simulink model "Admittace_Control"  (R2020a)
settings: Solver=FixedStepAuto  StartTime=0.0  StopTime=2  FixedStep=0.001  RelTol=1e-3  EnableMultiTasking=on
undefined symbols (not defined in the file or in its folder): X, Y, Z
libraries: sm_lib x79, nesl_utility x41, roblocks x8
(part 3 of 3)

== matlab function Admittace_Control/Exoskeleton/Subsystem/Admittance Control/xd+xe ==
  data: xyzkps0 input; xyzkps output; dxyzkps input
function xyzkps= add_compter(xyzkps0, dxyzkps)

xyzkps = zeros(1,6);
xyzkps(1)=xyzkps0(1)+dxyzkps(1);
xyzkps(2)=xyzkps0(2)+dxyzkps(2);
xyzkps(3)=xyzkps0(3)+dxyzkps(3);
%-------------
rpy=dxyzkps(4:6);
sx=sin(rpy(1));
cx=cos(rpy(1));
sy=sin(rpy(2));
cy=cos(rpy(2));
sz=sin(rpy(3));
cz=cos(rpy(3));
dR=[cy*cz  cz*sx*sy - cx*sz  sx*sz + cx*cz*sy;
	cy*sz  cx*cz + sx*sy*sz  cx*sy*sz - cz*sx;
	 -sy   cy*sx  cx*cy];

%-------------
rpy=xyzkps0(4:6);
sx=sin(rpy(1));
cx=cos(rpy(1));
sy=sin(rpy(2));
cy=cos(rpy(2));
sz=sin(rpy(3));
cz=cos(rpy(3));
R0=[cy*cz  cz*sx*sy - cx*sz  sx*sz + cx*cz*sy;
	cy*sz  cx*cz + sx*sy*sz  cx*sy*sz - cz*sx;
	 -sy   cy*sx  cx*cy];
R=dR*R0;
 
xyzkps(5)= atan2(-R(3,1),sqrt(R(1,1)*R(1,1)+R(2,1)*R(2,1))); 
        if (abs(abs(xyzkps(5)) - pi / 2.0) < 0.0000001)
                if (xyzkps(5) > 0) %pi/2
                    xyzkps(5) = pi / 2.0;
                    xyzkps(6) = 0.0;
                    xyzkps(4) = atan2(R(1,2),R(2,2));
                else%-pi/2
                    xyzkps(5) = -pi / 2.0;
                    xyzkps(6) = 0.0;
                    xyzkps(4) = -atan2(R(1,2), R(2,2));
                end
        else
                cp = cos(xyzkps(5));
                xyzkps(6) = atan2(R(2,1)/cp,R(1,1)/cp);
                xyzkps(4) = atan2(R(3,2)/cp, R(3,3)/cp);
        end


end

== matlab function Admittace_Control/Exoskeleton/Subsystem1/Admittance Control/jacobi ==
  data: Jn_Base input; dx output; dQ input
function dx = fcn(Jn_Base,dQ)
dx = Jn_Base*dQ;

== matlab function Admittace_Control/Exoskeleton/Subsystem1/Admittance Control/vel->pos ==
  data: dxe input; xe input; xe_targ output
function xe_targ   = vel_integral(dxe,xe)
%% parameter
xe_targ=zeros(1,6);
dt = 0.001;
dt_dxe=dxe*dt;
xe_targ(1)=xe(1)+dt_dxe(1);
xe_targ(2)=xe(2)+dt_dxe(2);
xe_targ(3)=xe(3)+dt_dxe(3);

%-----------等效转轴转姿态矩阵----------
eqaxis=dt_dxe(4:6);

A=norm(eqaxis);
if (A>1e-10)
axis=eqaxis./A;
sx=sin(A);cx=cos(A);v=1-cx;
dR=[axis(1)*axis(1)*v + cx	axis(1)*axis(2)*v - axis(3)*sx 	axis(1)*axis(3)*v + axis(2)*sx;
  axis(1)*axis(2)*v + axis(3)*sx 	axis(2)*axis(2)*v + cx 	 axis(2)*axis(3)*v - axis(1)*sx;
  axis(1)*axis(3)*v - axis(2)*sx 	axis(2)*axis(3)*v + axis(1)*sx  axis(3)*axis(3)*v + cx];
else
  dR=[1 0 0;
      0 1 0;
      0 0 1];
end

%-----------等效转轴转姿态矩阵----------
eqaxis=xe(4:6);
A=norm(eqaxis);
if (A>1e-10)
axis=eqaxis./A;
sx=sin(A);cx=cos(A);v=1-cx;
Re=[axis(1)*axis(1)*v + cx	axis(1)*axis(2)*v - axis(3)*sx 	axis(1)*axis(3)*v + axis(2)*sx;
  axis(1)*axis(2)*v + axis(3)*sx 	axis(2)*axis(2)*v + cx 	 axis(2)*axis(3)*v - axis(1)*sx;
  axis(1)*axis(3)*v - axis(2)*sx 	axis(2)*axis(3)*v + axis(1)*sx  axis(3)*axis(3)*v + cx];
else
  Re=[1 0 0;
      0 1 0;
      0 0 1];
end


R=dR*Re;%姿态叠加

%-----------姿态矩阵转固定角----------
xe_targ(5)= atan2(-R(3,1),sqrt(R(1,1)*R(1,1)+R(2,1)*R(2,1))); 
        if (abs(abs(xe_targ(5)) - pi / 2.0) < 0.0000001)
                if (xe_targ(5) > 0) %pi/2
                    xe_targ(5) = pi / 2.0;
                    xe_targ(6) = 0.0;
                    xe_targ(4) = atan2(R(1,2),R(2,2));
                else%-pi/2
                    xe_targ(5) = -pi / 2.0;
                    xe_targ(6) = 0.0;
                    xe_targ(4) = -atan2(R(1,2), R(2,2));
                end
        else
                cp = cos(xe_targ(5));
                xe_targ(6) = atan2(R(2,1)/cp,R(1,1)/cp);
                xe_targ(4) = atan2(R(3,2)/cp, R(3,3)/cp);
        end




end

== matlab function Admittace_Control/Exoskeleton/Subsystem1/Admittance Control/x-xd ==
  data: x input; xd input; xe output
function xe = Change(x,xd)
%% parameter
xe=zeros(1,6);
dt = 0.001;

V1 = [x(1)-xd(1),x(2)-xd(2),x(3)-xd(3) ];

p = x(4);
q = x(5);
r = x(6);
%% output
I= diag(ones(1,3));
%%
sx = sin(p);
cx = cos(p);
sy = sin(q);
cy = cos(q);
sz = sin(r);
cz = cos(r);
I(1,1) = cy*cz;			
I(1,2) = cz*sx*sy - cx*sz;	
I(1,3) = sx*sz + cx*cz*sy;
I(2,1) = cy*sz;	
I(2,2) = cx*cz + sx*sy*sz;			
I(2,3) = cx*sy*sz - cz*sx;
I(3,1) = -sy;	
I(3,2) = cy*sx;	
I(3,3) = cx*cy;

%%
pw = xd(4);
qw = xd(5);
rw = xd(6);
%% output
Iw= diag(ones(1,3));
%%
sxw = sin(pw);
cxw = cos(pw);
syw = sin(qw);
cyw = cos(qw);
szw = sin(rw);
czw = cos(rw);
Iw(1,1) = cyw*czw;			
Iw(1,2) = czw*sxw*syw - cxw*szw;	
Iw(1,3) = sxw*szw + cxw*czw*syw;
Iw(2,1) = cyw*szw;	
Iw(2,2) = cxw*czw + sxw*syw*szw;			
Iw(2,3) = cxw*syw*szw - czw*sxw;
Iw(3,1) = -syw;	
Iw(3,2) = cyw*sxw;	
Iw(3,3) = cxw*cyw;
V2=V1;
DI=I*Iw';
%%转换成等效转轴

cp=(DI(1,1)+DI(2,2)+DI(3,3)-1)/2.0;
if (cp>1-(1e-10))
    V2(1) = 0;
    V2(2) = 0;
    V2(3) = 0;
else
    if (cp<-1+(1e-10))
        V2(1) = sqrt( (DI(1,1)+1.0)/2);
        V2(2) = sqrt( (DI(2,2)+1.0)/2);
        V2(3) = sqrt( (DI(3,3)+1.0)/2);
        if ( DI(1,3)< 0)  
            V2(1) =- V2(1);
        end
        if ( DI(3,2)< 0)  
            V2(2) =- V2(2);
        end
        if (  V2(1)* V2(2)*DI(1,2) < 0)
            V2(1)=- V2(1);  % this last line can be necessary when z is 0
        end
            % z always >= 0
       % if z equal to zero
        V2(1) = V2(1)*pi;
        V2(2) = V2(2)*pi;
        V2(3) = V2(3)*pi;
    else
        Q=acos(cp);

        V2(1) = Q*0.5*(DI(3,2)-DI(2,3))/sin(Q);
        V2(2) = Q*0.5*(DI(1,3)-DI(3,1))/sin(Q);
        V2(3) = Q*0.5*(DI(2,1)-DI(1,2))/sin(Q);
    end
end
xe = [V1,V2];

end

== matlab function Admittace_Control/Exoskeleton/Subsystem1/Admittance Control/xd+xe ==
  data: xyzkps0 input; xyzkps output; dxyzkps input
function xyzkps= add_compter(xyzkps0, dxyzkps)

xyzkps = zeros(1,6);
xyzkps(1)=xyzkps0(1)+dxyzkps(1);
xyzkps(2)=xyzkps0(2)+dxyzkps(2);
xyzkps(3)=xyzkps0(3)+dxyzkps(3);
%-------------
rpy=dxyzkps(4:6);
sx=sin(rpy(1));
cx=cos(rpy(1));
sy=sin(rpy(2));
cy=cos(rpy(2));
sz=sin(rpy(3));
cz=cos(rpy(3));
dR=[cy*cz  cz*sx*sy - cx*sz  sx*sz + cx*cz*sy;
	cy*sz  cx*cz + sx*sy*sz  cx*sy*sz - cz*sx;
	 -sy   cy*sx  cx*cy];

%-------------
rpy=xyzkps0(4:6);
sx=sin(rpy(1));
cx=cos(rpy(1));
sy=sin(rpy(2));
cy=cos(rpy(2));
sz=sin(rpy(3));
cz=cos(rpy(3));
R0=[cy*cz  cz*sx*sy - cx*sz  sx*sz + cx*cz*sy;
	cy*sz  cx*cz + sx*sy*sz  cx*sy*sz - cz*sx;
	 -sy   cy*sx  cx*cy];
R=dR*R0;
 
xyzkps(5)= atan2(-R(3,1),sqrt(R(1,1)*R(1,1)+R(2,1)*R(2,1))); 
        if (abs(abs(xyzkps(5)) - pi / 2.0) < 0.0000001)
                if (xyzkps(5) > 0) %pi/2
                    xyzkps(5) = pi / 2.0;
                    xyzkps(6) = 0.0;
                    xyzkps(4) = atan2(R(1,2),R(2,2));
                else%-pi/2
                    xyzkps(5) = -pi / 2.0;
                    xyzkps(6) = 0.0;
                    xyzkps(4) = -atan2(R(1,2), R(2,2));
                end
        else
                cp = cos(xyzkps(5));
                xyzkps(6) = atan2(R(2,1)/cp,R(1,1)/cp);
                xyzkps(4) = atan2(R(3,2)/cp, R(3,3)/cp);
        end


end

== matlab function Admittace_Control/Exoskeleton/Subsystem1/Admittance Control/Admittance Control ==
  data: dxe input; xe input; ddxe output; Fe input; m_M parameter; m_B parameter; m_K parameter
function ddxe = fcn(dxe,xe,Fe,m_M, m_B, m_K)

%% control parameter
M = diag(m_M);
B = diag(m_B);
K = diag(m_K);

%% control
F_base=zeros(6,1);
F_base(1)=Fe(1);F_base(2)=Fe(2);F_base(3)=Fe(3);
F_base(4)=Fe(4);F_base(5)=Fe(5);F_base(6)=Fe(6);
dxe_base=zeros(6,1);
dxe_base(1)=dxe(1);dxe_base(2)=dxe(2);dxe_base(3)=dxe(3);
dxe_base(4)=dxe(4);dxe_base(5)=dxe(5);dxe_base(6)=dxe(6);
xe_base=zeros(6,1);
xe_base(1)=xe(1);xe_base(2)=xe(2);xe_base(3)=xe(3);
xe_base(4)=xe(4);xe_base(5)=xe(5);xe_base(6)=xe(6);
tmp=(F_base-B*dxe_base-K*xe_base);
if (norm(tmp)>1e-10)
    ddxe = M^(-1)*(F_base-B*dxe_base-K*xe_base);
else
    ddxe=zeros(6,1);
end

end

== matlab function Admittace_Control/Exoskeleton/Subsystem1/pulse ==
  data: in input; out output
function out  = pulse_set(in)

persistent out_;
if isempty(out_)
out_ = 0;
end
persistent flag;
if isempty(flag)
flag = 0;
end

if ((1==in)&&(0==flag))
   out_=1;
   flag=1;
end

if (0==in)
    flag=0;
end

out=out_;
out_=0;
end

== matlab function Admittace_Control/Exoskeleton/Subsystem1/数值微分 ==
  data: out output; in input; set input
function out  = diff(in,set)
persistent in_;
if isempty(in_)
in_ = in;
end
if (1==set)
   in_=in; 
end


out=(in-in_).*1000;

in_=in;


end

== matlab function Admittace_Control/Exoskeleton/Subsystem/pulse ==
  data: in input; out output
function out  = pulse_set(in)

persistent out_;
if isempty(out_)
out_ = 0;
end
persistent flag;
if isempty(flag)
flag = 0;
end

if ((1==in)&&(0==flag))
   out_=1;
   flag=1;
end

if (0==in)
    flag=0;
end

out=out_;
out_=0;
end

== matlab function Admittace_Control/Exoskeleton/Subsystem/数值微分 ==
  data: out output; in input; set input
function out  = diff(in,set)
persistent in_;
if isempty(in_)
in_ = in;
end
if (1==set)
   in_=in; 
end


out=(in-in_).*1000;

in_=in;


end

== matlab function Admittace_Control/Exoskeleton/Subsystem/法兰坐标系下力矩转换为基坐标系下 ==
  data: Fsensor input; Fe output; T input
function Fe = fcn(Fsensor,T)
Tchange = T;
T33 = Tchange(1:3,1:3);
T330 = zeros(3,3);
T66= [T33 T330;
    T330 T33];
Fe = T66*Fsensor;

== matlab function Admittace_Control/Exoskeleton/Subsystem1/法兰坐标系下力矩转换为基坐标系下 ==
  data: Fsensor input; Fe output; T input
function Fe = fcn(Fsensor,T)
Tchange = T;
T33 = Tchange(1:3,1:3);
T330 = zeros(3,3);
T66= [T33 T330;
    T330 T33];
Fe = T66*Fsensor;

== matlab function Admittace_Control/Exoskeleton/XB FK1/DH-CC1 ==
  data: KPS44 input; KPS6 output
function KPS6  = FK(KPS44)
%% parameter
rpy = zeros(1,3);
eps = 0.000001;
%% input 
T=[1 0 0 0;0 1 0 0; 0 0 1 0];
G=KPS44;
H =T * ( G * [0;0;0;1]);
%%
rpy(2) = atan2(-KPS44(3,1),sqrt(KPS44(1,1)*KPS44(1,1)+KPS44(2,1)*KPS44(2,1)));
if (abs(abs(rpy(2)) - pi / 2.0) < eps)
	if (rpy(2) > 0) 
        rpy(2) = pi / 2.0;
        rpy(3) = 0.0;
        rpy(1) = atan2(KPS44(1,2),KPS44(2,2));
    else
    rpy(2) = -pi / 2.0;
	rpy(3) = 0.0;
	rpy(1) = -atan2(KPS44(1,2), KPS44(2,2));
	end
else
	cp = cos(rpy(2));
	rpy(3) = atan2(KPS44(2,1)/cp,KPS44(1,1)/cp);
	rpy(1) = atan2(KPS44(3,2)/cp, KPS44(3,3)/cp);
end
KPS6 = [H' rpy]; 
end

== matlab function Admittace_Control/Exoskeleton/Subsystem1/Admittance Control/XB FK/DH-CC1 ==
  data: KPS44 input; KPS6 output
function KPS6  = FK(KPS44)
%% parameter
rpy = zeros(1,3);
eps = 0.000001;
%% input 
T=[1 0 0 0;0 1 0 0; 0 0 1 0];
G=KPS44;
H =T * ( G * [0;0;0;1]);
%%
rpy(2) = atan2(-KPS44(3,1),sqrt(KPS44(1,1)*KPS44(1,1)+KPS44(2,1)*KPS44(2,1)));
if (abs(abs(rpy(2)) - pi / 2.0) < eps)
	if (rpy(2) > 0) 
        rpy(2) = pi / 2.0;
        rpy(3) = 0.0;
        rpy(1) = atan2(KPS44(1,2),KPS44(2,2));
    else
    rpy(2) = -pi / 2.0;
	rpy(3) = 0.0;
	rpy(1) = -atan2(KPS44(1,2), KPS44(2,2));
	end
else
	cp = cos(rpy(2));
	rpy(3) = atan2(KPS44(2,1)/cp,KPS44(1,1)/cp);
	rpy(1) = atan2(KPS44(3,2)/cp, KPS44(3,3)/cp);
end
KPS6 = [H' rpy]; 
end

== matlab function Admittace_Control/Exoskeleton/Subsystem/Admittance Control/Admittance Control ==
  data: dxe input; xe input; ddxe output; Fe input; m_M parameter; m_B parameter; m_K parameter
function ddxe = fcn(dxe,xe,Fe,m_M, m_B, m_K)

%% control parameter
M = diag(m_M);
B = diag(m_B);
K = diag(m_K);

%% control
F_base=zeros(6,1);
F_base(1)=Fe(1);F_base(2)=Fe(2);F_base(3)=Fe(3);
F_base(4)=Fe(4);F_base(5)=Fe(5);F_base(6)=Fe(6);
dxe_base=zeros(6,1);
dxe_base(1)=dxe(1);dxe_base(2)=dxe(2);dxe_base(3)=dxe(3);
dxe_base(4)=dxe(4);dxe_base(5)=dxe(5);dxe_base(6)=dxe(6);
xe_base=zeros(6,1);
xe_base(1)=xe(1);xe_base(2)=xe(2);xe_base(3)=xe(3);
xe_base(4)=xe(4);xe_base(5)=xe(5);xe_base(6)=xe(6);
tmp=(F_base-B*dxe_base-K*xe_base);
if (norm(tmp)>1e-10)
    ddxe = M^(-1)*(F_base-B*dxe_base-K*xe_base);
else
    ddxe=zeros(6,1);
end

end

== matlab function Admittace_Control/Exoskeleton/Subsystem1/Admittance Control/XB04 IK/DH-IK-CC ==
  data: KPS6 input; KPS44 output
function KPS44  = IK(KPS6)
%% input 
x = KPS6(1);
y = KPS6(2);
z = KPS6(3);
p = KPS6(4);
q = KPS6(5);
r = KPS6(6);
%% output
I= diag(ones(1,4));
%%
sx = sin(p);
cx = cos(p);
sy = sin(q);
cy = cos(q);
sz = sin(r);
cz = cos(r);
I(1,1) = cy*cz;			
I(1,2) = cz*sx*sy - cx*sz;	
I(1,3) = sx*sz + cx*cz*sy;
I(2,1) = cy*sz;	
I(2,2) = cx*cz + sx*sy*sz;			
I(2,3) = cx*sy*sz - cz*sx;
I(3,1) = -sy;	
I(3,2) = cy*sx;	
I(3,3) = cx*cy;
I(1,4) = x ;
I(2,4) = y ;
I(3,4) = z ;
I(4,4) = 1 ; 


%%
KPS44 = I;
end

== matlab function Admittace_Control/Exoskeleton/Subsystem/Admittance Control/XB FK/DH-CC1 ==
  data: KPS44 input; KPS6 output
function KPS6  = FK(KPS44)
%% parameter
rpy = zeros(1,3);
eps = 0.000001;
%% input 
T=[1 0 0 0;0 1 0 0; 0 0 1 0];
G=KPS44;
H =T * ( G * [0;0;0;1]);
%%
rpy(2) = atan2(-KPS44(3,1),sqrt(KPS44(1,1)*KPS44(1,1)+KPS44(2,1)*KPS44(2,1)));
if (abs(abs(rpy(2)) - pi / 2.0) < eps)
	if (rpy(2) > 0) 
        rpy(2) = pi / 2.0;
        rpy(3) = 0.0;
        rpy(1) = atan2(KPS44(1,2),KPS44(2,2));
    else
    rpy(2) = -pi / 2.0;
	rpy(3) = 0.0;
	rpy(1) = -atan2(KPS44(1,2), KPS44(2,2));
	end
else
	cp = cos(rpy(2));
	rpy(3) = atan2(KPS44(2,1)/cp,KPS44(1,1)/cp);
	rpy(1) = atan2(KPS44(3,2)/cp, KPS44(3,3)/cp);
end
KPS6 = [H' rpy]; 
end

== matlab function Admittace_Control/Exoskeleton/Subsystem/Admittance Control/XB04 IK/DH-IK-CC ==
  data: KPS6 input; KPS44 output
function KPS44  = IK(KPS6)
%% input 
x = KPS6(1);
y = KPS6(2);
z = KPS6(3);
p = KPS6(4);
q = KPS6(5);
r = KPS6(6);
%% output
I= diag(ones(1,4));
%%
sx = sin(p);
cx = cos(p);
sy = sin(q);
cy = cos(q);
sz = sin(r);
cz = cos(r);
I(1,1) = cy*cz;			
I(1,2) = cz*sx*sy - cx*sz;	
I(1,3) = sx*sz + cx*cz*sy;
I(2,1) = cy*sz;	
I(2,2) = cx*cz + sx*sy*sz;			
I(2,3) = cx*sy*sz - cz*sx;
I(3,1) = -sy;	
I(3,2) = cy*sx;	
I(3,3) = cx*cy;
I(1,4) = x ;
I(2,4) = y ;
I(3,4) = z ;
I(4,4) = 1 ; 


%%
KPS44 = I;
end

== matlab function Admittace_Control/Exoskeleton/XB FK/DH-CC1 ==
  data: KPS44 input; KPS6 output
function KPS6  = FK(KPS44)
%% parameter
rpy = zeros(1,3);
eps = 0.000001;
%% input 
T=[1 0 0 0;0 1 0 0; 0 0 1 0];
G=KPS44;
H =T * ( G * [0;0;0;1]);
%%
rpy(2) = atan2(-KPS44(3,1),sqrt(KPS44(1,1)*KPS44(1,1)+KPS44(2,1)*KPS44(2,1)));
if (abs(abs(rpy(2)) - pi / 2.0) < eps)
	if (rpy(2) > 0) 
        rpy(2) = pi / 2.0;
        rpy(3) = 0.0;
        rpy(1) = atan2(KPS44(1,2),KPS44(2,2));
    else
    rpy(2) = -pi / 2.0;
	rpy(3) = 0.0;
	rpy(1) = -atan2(KPS44(1,2), KPS44(2,2));
	end
else
	cp = cos(rpy(2));
	rpy(3) = atan2(KPS44(2,1)/cp,KPS44(1,1)/cp);
	rpy(1) = atan2(KPS44(3,2)/cp, KPS44(3,3)/cp);
end
KPS6 = [H' rpy]; 
end

== matlab function Admittace_Control/Exoskeleton/Subsystem/Admittance Control/XB04 IK/MATLAB Function ==
  data: T input; q output
function q= fcn(T)
%theta-offset
offset1 = 0;
offset2 = pi/2-atan(0.23966/0.28189);
offset3 = pi/2-atan(0.23966/0.28189)+atan(0.15989/0.31135);
offset4 = -atan(0.15989/0.31135);
%%DH
d1 = -0.097;
a3 = -sqrt(0.23966^2+0.28189^2);
a4 = -sqrt(-0.15989^2+0.31135^2);
%%theta1
  theta1 = atan2(T(1,3),-T(2,3));
%%theta3
  equ1 = T(1,4)^2 + T(2,4)^2;
  equ2 = (T(3,4)-d1)^2;
  equ3 = equ1 + equ2;
  c3   = (equ3 - a3^2 - a4^2)/(2*a3*a4);
%   s3   = sqrt(1-c3^2);
  if 1-c3^2 < 1e-20
      s3 = 0;
  else
      s3   = sqrt(1-c3^2);
  end
  theta3 = atan2(s3,c3);
  
%%theta2
  
  x = (T(1,4)^2+T(2,4)^2)^0.5;
  y = T(3,4)-d1;
  if T(1,4) < 0
      x = -x;
  end
  k1 = (a4*cos(theta3)+a3);
  k2 = -sin(theta3)*a4;
  theta2 = atan2(y,x)+ atan2(k2,k1);
%   theta2 = -theta2;
  
%%theta4
  phi = atan2(T(3,1),T(3,2));
  theta4 = phi - theta2 - theta3;
  q = [0,theta1,theta2,theta3,theta4];

== matlab function Admittace_Control/Exoskeleton/Subsystem/Admittance Control/acc->vel ==
  data: ddxe input; dxe input; dxe_targ output
function dxe_targ   = acc_integral(ddxe,dxe)
%% parameter
dt = 0.001;
dxe_targ=zeros(1,6);
dt_ddxe=ddxe*dt;
dxe_targ(1)=dxe(1)+dt_ddxe(1);
dxe_targ(2)=dxe(2)+dt_ddxe(2);
dxe_targ(3)=dxe(3)+dt_ddxe(3);
dxe_targ(4)=dxe(4)+dt_ddxe(4);
dxe_targ(5)=dxe(5)+dt_ddxe(5);
dxe_targ(6)=dxe(6)+dt_ddxe(6);


end

== matlab function Admittace_Control/Exoskeleton/Subsystem/Admittance Control/jacobi ==
  data: Jn_Base input; dx output; dQ input
function dx = fcn(Jn_Base,dQ)
dx = Jn_Base*dQ;

== matlab function Admittace_Control/Exoskeleton/Subsystem/Admittance Control/vel->pos ==
  data: dxe input; xe input; xe_targ output
function xe_targ   = vel_integral(dxe,xe)
%% parameter
xe_targ=zeros(1,6);
dt = 0.001;
dt_dxe=dxe*dt;
xe_targ(1)=xe(1)+dt_dxe(1);
xe_targ(2)=xe(2)+dt_dxe(2);
xe_targ(3)=xe(3)+dt_dxe(3);

%-----------等效转轴转姿态矩阵----------
eqaxis=dt_dxe(4:6);

A=norm(eqaxis);
if (A>1e-10)
axis=eqaxis./A;
sx=sin(A);cx=cos(A);v=1-cx;
dR=[axis(1)*axis(1)*v + cx	axis(1)*axis(2)*v - axis(3)*sx 	axis(1)*axis(3)*v + axis(2)*sx;
  axis(1)*axis(2)*v + axis(3)*sx 	axis(2)*axis(2)*v + cx 	 axis(2)*axis(3)*v - axis(1)*sx;
  axis(1)*axis(3)*v - axis(2)*sx 	axis(2)*axis(3)*v + axis(1)*sx  axis(3)*axis(3)*v + cx];
else
  dR=[1 0 0;
      0 1 0;
      0 0 1];
end

%-----------等效转轴转姿态矩阵----------
eqaxis=xe(4:6);
A=norm(eqaxis);
if (A>1e-10)
axis=eqaxis./A;
sx=sin(A);cx=cos(A);v=1-cx;
Re=[axis(1)*axis(1)*v + cx	axis(1)*axis(2)*v - axis(3)*sx 	axis(1)*axis(3)*v + axis(2)*sx;
  axis(1)*axis(2)*v + axis(3)*sx 	axis(2)*axis(2)*v + cx 	 axis(2)*axis(3)*v - axis(1)*sx;
  axis(1)*axis(3)*v - axis(2)*sx 	axis(2)*axis(3)*v + axis(1)*sx  axis(3)*axis(3)*v + cx];
else
  Re=[1 0 0;
      0 1 0;
      0 0 1];
end


R=dR*Re;%姿态叠加

%-----------姿态矩阵转固定角----------
xe_targ(5)= atan2(-R(3,1),sqrt(R(1,1)*R(1,1)+R(2,1)*R(2,1))); 
        if (abs(abs(xe_targ(5)) - pi / 2.0) < 0.0000001)
                if (xe_targ(5) > 0) %pi/2
                    xe_targ(5) = pi / 2.0;
                    xe_targ(6) = 0.0;
                    xe_targ(4) = atan2(R(1,2),R(2,2));
                else%-pi/2
                    xe_targ(5) = -pi / 2.0;
                    xe_targ(6) = 0.0;
                    xe_targ(4) = -atan2(R(1,2), R(2,2));
                end
        else
                cp = cos(xe_targ(5));
                xe_targ(6) = atan2(R(2,1)/cp,R(1,1)/cp);
                xe_targ(4) = atan2(R(3,2)/cp, R(3,3)/cp);
        end




end
